simulink model "Observador_ex1"  (R2021a)
settings: Solver=VariableStepAuto  StartTime=0.0  StopTime=5  RelTol=1e-3
values from neighbouring files (symbols this model uses):
  A = [1 -1 0.01 0.12]    [Real_Esta_Disc_Ref.m]    (also in Routh_Hurwitz.m = [0 1 0;0 0 1;-160 -56 -14]; Smulacro_Parcial_Final.m = matrizA; observador_estados_ex1.m = [-20 1 ;-1 0]; tercer_orden.m = 1)
  b = [5 1 2]    [Realimentacion_Acker.m]    (also in Resumen_PrimerCorte_obsContrRouth.m = [1]; RouthPrueba.m = [rand(1,((l-1)/2)),0]; observador_estados_ex1.m = [1; 0])
  c = zeros(l,l1)    [RouthPrueba.m]    (also in observador_estados_ex1.m = [0 1])
  l = length(e)    [RouthPrueba.m]    (also in observador_estados_ex1.m = k')
settings Model: Creator=Sergio  LastModifiedBy=Sergio
settings SolverCC: AlgebraicLoopSolver=TrustRegion
settings DebuggingCC: SFMachineParentedDataDiag=warning

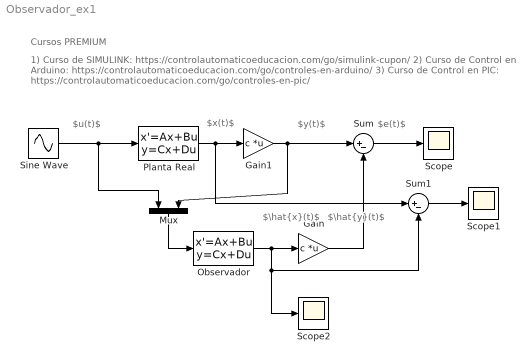
== system Observador_ex1 ==
  note: Cursos PREMIUM
  note: 1) Curso de SIMULINK: https://controlautomaticoeducacion.com/go/simulink-cupon/
      | 2) Curso de Control en Arduino: https://controlautomaticoeducacion.com/go/controles-en-arduino/
      | 3) Curso de Control en PIC: https://controlautomaticoeducacion.com/go/controles-en-pic/
  note: $\hat{y}(t)$
  note: $y(t)$
  note: $u(t)$
  note: $e(t)$
  note: $\hat{x}(t)$
  note: $x(t)$
  Gain : Gain  Gain=c  Multiplication=Matrix(K*u)
  Gain1 : Gain  Gain=c  Multiplication=Matrix(K*u)
  Mux : Mux  Inputs=2
  Observador : StateSpace  A=A-l*c  B=[b,l]  C=eye(2)  D=zeros(2)  InitialCondition=[0; 0]
  Planta Real : StateSpace  A=A  B=b  C=eye(2)  D=[0 0]'  InitialCondition=[1 0]
  Scope : Scope
  Scope1 : Scope
  Scope2 : Scope
  Sine Wave : Sin  Frequency=0.5  SampleTime=0
  Sum : Sum  Inputs=|+-
  Sum1 : Sum  Inputs=|+-
  wires:
  Mux/1 -> Observador/1
  Planta Real/1 -> Sum1/1, Gain1/1
  Sine Wave/1 -> Mux/1, Planta Real/1
  Observador/1 -> Scope2/1, Sum1/2, Gain/1
  Gain/1 -> Sum/2
  Sum/1 -> Scope/1
  Gain1/1 -> Mux/2, Sum/1
  Sum1/1 -> Scope1/1
